simulink model "window_in_window_out_with_margin"  (R2019b)
settings: Solver=VariableStepAuto  StartTime=0.0  StopTime=128  RelTol=1e-3
InitFcn:
  | xmcCheckSlxPath(bdroot);
undefined symbols (not defined in the file): xc7vx485tffg1157
libraries: ModelComposer x3, dspsrcs4 x1
settings Model: Creator=viswanad  LastModifiedBy=abehbood
settings SFSimCC: CustomCodeUndefinedFunction=UseInterfaceOnly

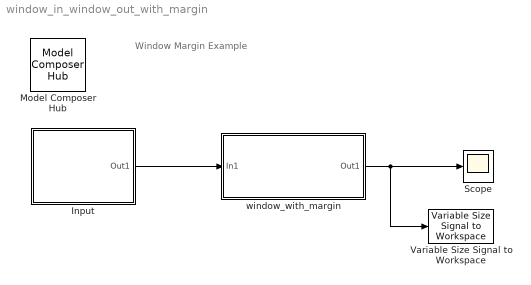
== system window_in_window_out_with_margin ==
  note: Window Margin Example
  Input : Subsystem
  Model Composer Hub : ModelComposer/Model Composer Hub  CodeGeneration=off  SubsystemName=window_with_margin  TargetDirectory=./code  ExportType=AI Engines  IpVendor=xilinx.com  IpLibrary=hls  IpVersion=1.0  IpHWLanguage=Verilog  AieCompilerOptions={}  CreateTestbench=on  TestbenchStackSize=10  RunAieSim=on  AieSimTimeout=50000  LaunchVitisAnalyzer=off  RunX86Sim=off  X86SimTimeout=10  ProjDevice=xc7vx485tffg1157-1  ProjDevicePart=xc7vx485tffg1157-1  SamplePeriod=-1  ClockFrequency=200  DataPathParallelism=1
  Scope : Scope
  Variable Size Signal to Workspace : ModelComposer/Variable Size Signal to Workspace  VariableNameMask=simout
  window_with_margin : Subsystem
  wires:
  window_with_margin/1(Out1) -> Variable Size Signal to Workspace/1, Scope/1
  Input/1(Out1) -> window_with_margin/1(In1)

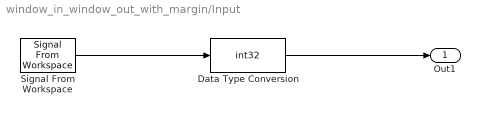
== system window_in_window_out_with_margin/Input ==
  Data Type Conversion : DataTypeConversion  OutDataTypeStr=int32
  Signal From Workspace : dspsrcs4/Signal From Workspace  X=1:128  Ts=24/16  nsamps=16  OutputAfterFinalValue=Setting to zero  ignoreOrWarnInputAndFrameLengths=off  OutputFrames=off
  Out1 : Outport  VectorParamsAs1DForOutWhenUnconnected=off
  wires:
  Signal From Workspace/1 -> Data Type Conversion/1
  Data Type Conversion/1 -> Out1/1

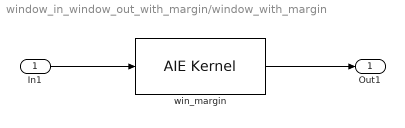
== system window_in_window_out_with_margin/window_with_margin ==
  In1 : Inport
  win_margin : ModelComposer/AIE Kernel  PortAttributesTable={ 'Input', 'inw', 'input_window_int32 *', '16', '8', 'auto', ''; 'Output', 'outw', 'output_window_int32 *', '24', '', 'auto', '' }  PortAttributesEnablement={'off', 'off', 'off', 'on', 'on', 'on', 'off';'off', 'off', 'off', 'on', 'off', 'on', 'off'}  FormalArgDecls={'input_window_int32 * inw', 'output_window_int32 * outw'}  PortWindowSizes={1.600000000000000000e+01; 2.400000000000000000e+01}  PortWindowMargins={8.000000000000000000e+00; 0.000000000000000000e+00}  PortSynchronicities={'auto'; 'auto'}  PortSignalSizes={0.000000000000000000e+00; 0.000000000000000000e+00}  SimLibPath=''  FunctionTabVisible=on  FunctionDescription=void win_margin(input_window_int32 * inw, output_window_int32 * outw)  KernelHeaderFile=src/kernels/window_in_window_out_margin.h  KernelFunction=win_margin  KernelFunctionSelect=<empty>  KernelSourceFile=src/kernels/window_in_window_out_margin.cc  KernelSearchPaths={}  PreProcOptions={}  CoreRuntimeRatio=0.9  KernelLocSpec=off  ColRowLocation=[0 0]
  Out1 : Outport  VectorParamsAs1DForOutWhenUnconnected=off
  wires:
  In1/1 -> win_margin/1
  win_margin/1 -> Out1/1
